simulink model "MPC2018a"  (R2019b)
settings: Solver=FixedStepAuto  StartTime=0.0  StopTime=80  FixedStep=0.05  RelTol=1e-3
InitFcn:
  | startPose=[0,0,48]
StopFcn:
  | load('NewBaiYunPathDown6_13.mat')
  | n=1;
  | x0=0;
  | y0=0;
  | lng0 = BaiYunEmpty(2,1);
  | lat0 = BaiYunEmpty(1,1);
  | x1=[];
  | y1=[];
  | head=[];
  | nn = length(BaiYunEmpty(1,:));
  | while (n<nn)
  | lng2 = BaiYunEmpty(2,n);
  | lat2 = BaiYunEmpty(1,n);
  | head2 = BaiYunEmpty(3,n);
  | temp_x=(lng2-lng0)*111700*cos(lat2/180*pi);
  | temp_y=(lat2-lat0)*111700;
  | x1(n) = x0 + temp_x;
  | y1(n) = y0 + temp_y;
  | head(n)=head2;
  | n = n+1;
  | end
  | figure(1);
  | plot(x1,y1,'+r',out.v2(:,1),out.v2(:,2),'+k',out.v3(:,1),out.v3(:,2),'+b');
libraries: simulink x21, simulink_extras x4, drivingvehiclecontroller x2, vehdynlibsteering x2, autolibshared x2
(part 1 of 2)
settings Model: NumberOfSteps=10  SnapshotBufferSize=100  Creator=hurui  LastModifiedBy=HL
settings SolverCC: AlgebraicLoopSolver=LineSearch
settings DataIOCC: SaveFormat=StructureWithTime
settings OptimizationCC: BlockReduction=off  UseDivisionForNetSlopeComputation=on  BufferReuse=off
settings DebuggingCC: AlgebraicLoopMsg=none  UnconnectedInputMsg=none  UnconnectedOutputMsg=none  UnconnectedLineMsg=none  UnderSpecifiedDimensionMsg=warning
settings SFSimCC: SimParseCustomCode=off

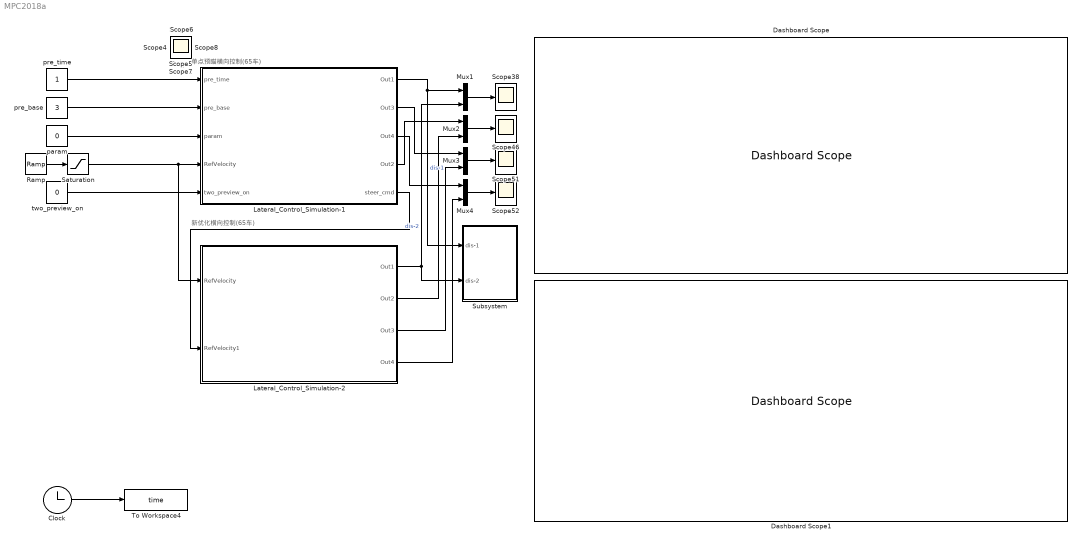
== system MPC2018a ==
  note: 单点预瞄横向控制(65车)
  note: 新优化横向控制(65车)
  Clock : Clock
  Dashboard Scope : DashboardScope
  Dashboard Scope1 : DashboardScope
  Lateral_Control_Simulation-1 : Subsystem
  Lateral_Control_Simulation-2 : Subsystem
  Mux{1..4} (4 alike) : Mux  Inputs=2
  Ramp : simulink/Sources/Ramp  slope=1  start=0  InitialOutput=0
  Saturation : Saturate  UpperLimit=15  LowerLimit=0
  Scope{,1..8,38,46,51..52} (13 alike) : Scope
  Subsystem : Subsystem
  To Workspace4 : ToWorkspace  VariableName=time  SampleTime=-1
      settings: Save2DSignal=2-D array (concatenate along first dimension)
  param : Constant  Value=0  OutDataTypeStr=single
  pre_base : Constant  Value=3  OutDataTypeStr=single
  pre_time : Constant  OutDataTypeStr=single
  two_preview_on : Constant  Value=0  OutDataTypeStr=single
  wires:
  Lateral_Control_Simulation-1/1(Out1) -> Subsystem/1(dis-1), Mux1/1  "dis-1"
  Lateral_Control_Simulation-2/1(Out1) -> Mux1/2, Subsystem/2(dis-2)  "dis-2"
  Mux1/1 -> Scope38/1
  Lateral_Control_Simulation-1/4(Out2) -> Mux2/1
  Lateral_Control_Simulation-2/2(Out2) -> Mux2/2
  Mux2/1 -> Scope46/1
  pre_time/1 -> Lateral_Control_Simulation-1/1(pre_time)
  pre_base/1 -> Lateral_Control_Simulation-1/2(pre_base)
  param/1 -> Lateral_Control_Simulation-1/3(param)
  Saturation/1 -> Lateral_Control_Simulation-1/4(RefVelocity), Lateral_Control_Simulation-2/1(RefVelocity)
  two_preview_on/1 -> Lateral_Control_Simulation-1/5(two_preview_on)
  Clock/1 -> To Workspace4/1
  Ramp/1 -> Saturation/1
  Lateral_Control_Simulation-1/2(Out3) -> Mux3/1
  Lateral_Control_Simulation-2/3(Out3) -> Mux3/2
  Lateral_Control_Simulation-1/3(Out4) -> Mux4/1
  Lateral_Control_Simulation-2/4(Out4) -> Mux4/2
  Mux3/1 -> Scope51/1
  Mux4/1 -> Scope52/1
  Lateral_Control_Simulation-1/5(steer_cmd) -> Lateral_Control_Simulation-2/2(RefVelocity1)

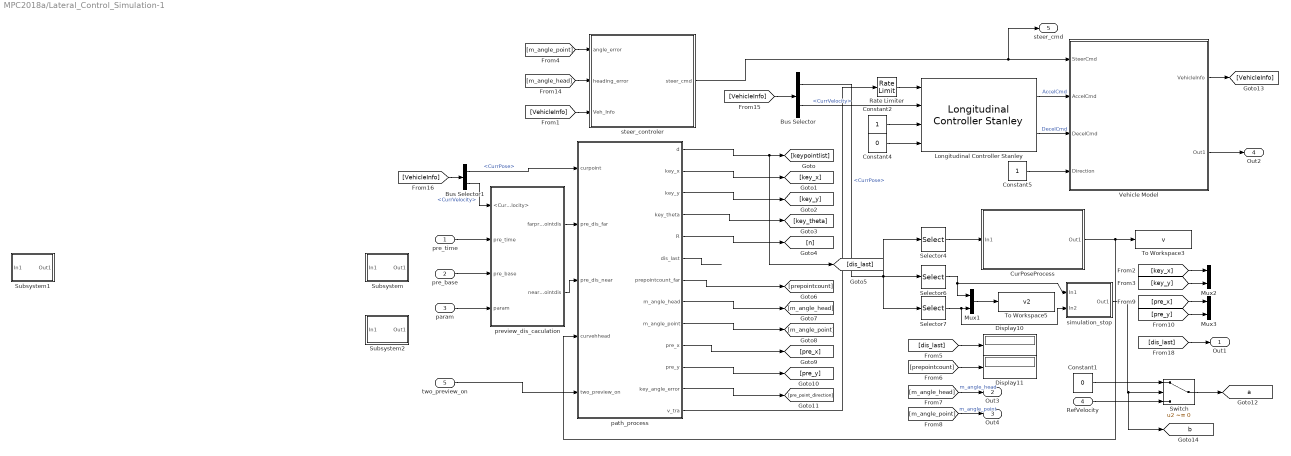
== system MPC2018a/Lateral_Control_Simulation-1 ==
  pre_time : Inport
  pre_base : Inport  Port=2
  param : Inport  Port=3
  RefVelocity : Inport  Port=4
  two_preview_on : Inport  Port=5
  Bus Selector : BusSelector  OutputSignals=CurrPose,CurrVelocity
  Bus Selector1 : BusSelector  OutputSignals=CurrPose,CurrVelocity
  Constant1 : Constant  Value=0
  Constant2 : Constant
  Constant4 : Constant  Value=0
  Constant5 : Constant
  CurPoseProcess : Subsystem
  Display10 : Display
  Display11 : Display
  Longitudinal Controller Stanley : drivingvehiclecontroller/Longitudinal Controller Stanley  Kp=2.5  Ki=1  SampleTime=0.05  MaxAcceleration=3  MaxDeceleration=25
      settings: SourceProductBaseCode=DR
  Mux1 : Mux  Inputs=2
  Mux2 : Mux  Inputs=2
  Mux3 : Mux  Inputs=2
  Rate Limiter : RateLimiter  SampleTimeMode=inherited
  Selector4 : Selector  InputPortWidth=3  IndexOptions=Index vector (dialog)  Indices=[3]  OutputSizes=1
  Selector6 : Selector  InputPortWidth=3  IndexOptions=Index vector (dialog)  Indices=[1]  OutputSizes=1
  Selector7 : Selector  InputPortWidth=3  IndexOptions=Index vector (dialog)  Indices=[2]  OutputSizes=1
  Subsystem : Subsystem
  Subsystem1 : Subsystem
  Subsystem2 : Subsystem
  Switch : Switch  Criteria=u2 ~= 0
  To Workspace3 : ToWorkspace  VariableName=v  SampleTime=-1
      settings: Save2DSignal=2-D array (concatenate along first dimension)
  To Workspace5 : ToWorkspace  VariableName=v2  SampleTime=-1
      settings: Save2DSignal=2-D array (concatenate along first dimension)
  Vehicle Model : Subsystem
  path_process : MATLAB Function  TreatAsAtomicUnit=on  VariantControl=(default)
  preview_dis_caculation : Subsystem
  simulation_stop : Subsystem
  steer_controler : Subsystem
  Out1 : Outport
  Out3 : Outport  Port=2
  Out4 : Outport  Port=3
  Out2 : Outport  Port=4
  steer_cmd : Outport  Port=5
  tag scope: a=global, b=global
  wires:
  pre_time/1 -> preview_dis_caculation/2(pre_time)
  pre_base/1 -> preview_dis_caculation/3(pre_base)
  param/1 -> preview_dis_caculation/4(param)
  [dis_last] -> Out1/1
  path_process/8(m_angle_head) -> [m_angle_head]
  Bus Selector/1 -> Selector4/1, Selector7/1, Selector6/1  "<CurrPose>"
  [VehicleInfo] -> Bus Selector1/1
  Mux1/1 -> To Workspace5/1
  Constant2/1 -> Longitudinal Controller Stanley/3
  path_process/6(dis_last) -> ?
  preview_dis_caculation/1(farprepointdis) -> path_process/2(pre_dis_far)
  Longitudinal Controller Stanley/2 -> Vehicle Model/3(DecelCmd)  "DecelCmd"
  Bus Selector/2 -> Longitudinal Controller Stanley/2  "<CurrVelocity>"
  path_process/4(key_theta) -> [key_theta]
  [VehicleInfo] -> steer_controler/3(Veh_Info)
  Bus Selector1/1 -> path_process/1(curpoint)  "<CurrPose>"
  Selector6/1 -> Mux1/1, simulation_stop/1(In1)
  Constant4/1 -> Longitudinal Controller Stanley/4
  Constant5/1 -> Vehicle Model/4(Direction)
  preview_dis_caculation/2(nearprepointdis) -> path_process/3(pre_dis_near)
  [m_angle_head] -> Out3/1  "m_angle_head"
  path_process/7(prepointcount_far) -> [prepointcount]
  Selector7/1 -> simulation_stop/2(In2), Mux1/2
  path_process/12(key_angle_error) -> [pre_point_direction]
  path_process/10(pre_x) -> [pre_x]
  path_process/2(key_x) -> [key_x]
  [pre_y] -> Mux3/2
  steer_controler/1(steer_cmd) -> steer_cmd/1, Vehicle Model/1(SteerCmd)
  [key_x] -> Mux2/1
  Longitudinal Controller Stanley/1 -> Vehicle Model/2(AccelCmd)  "AccelCmd"
  path_process/3(key_y) -> [key_y]
  Bus Selector1/2 -> preview_dis_caculation/1(<CurrVelocity>)  "<CurrVelocity>"
  path_process/9(m_angle_point) -> [m_angle_point]
  [VehicleInfo] -> Bus Selector/1
  [pre_x] -> Mux3/1
  [key_y] -> Mux2/2
  [m_angle_head] -> steer_controler/2(heading_error)
  [dis_last] -> Display10/1
  [m_angle_point] -> Out4/1  "m_angle_point"
  [m_angle_point] -> steer_controler/1(angle_error)
  path_process/11(pre_y) -> [pre_y]
  [prepointcount] -> Display11/1
  path_process/5(R) -> [n]
  Vehicle Model/1(VehicleInfo) -> [VehicleInfo]
  RefVelocity/1 -> Switch/3
  Selector4/1 -> CurPoseProcess/1(In1)
  CurPoseProcess/1(Out1) -> path_process/4(curvehhead), To Workspace3/1
  two_preview_on/1 -> path_process/5(two_preview_on)
  Vehicle Model/2(Out1) -> Out2/1
  simulation_stop/1(Out1) -> [b], Switch/2
  Constant1/1 -> Switch/1
  Switch/1 -> [a]
  Rate Limiter/1 -> Longitudinal Controller Stanley/1
  path_process/13(v_tra) -> Rate Limiter/1
  path_process/1(d) -> [dis_last], [keypointlist]

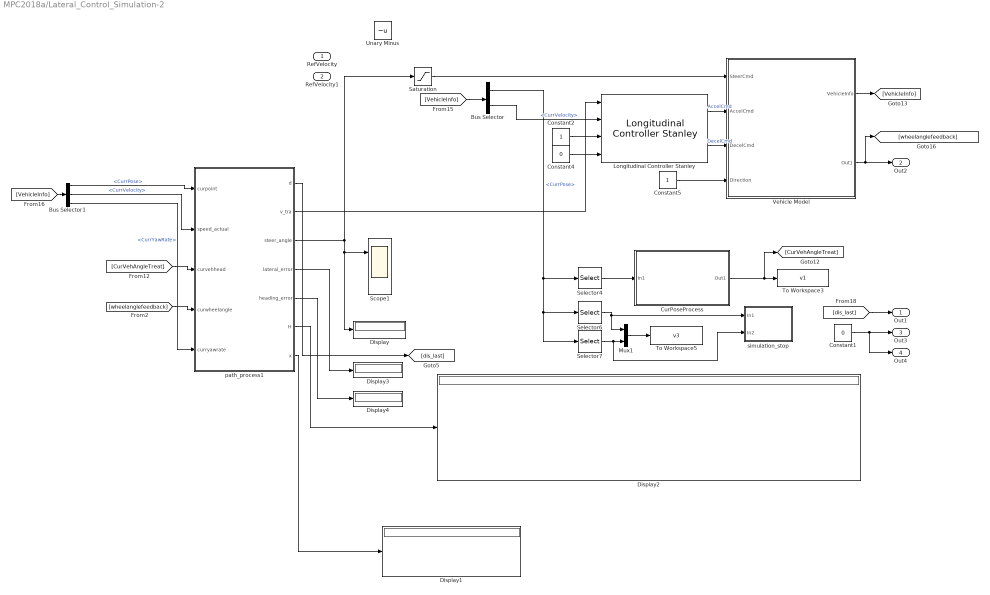
== system MPC2018a/Lateral_Control_Simulation-2 ==
  RefVelocity : Inport
  RefVelocity1 : Inport  Port=2
  Bus Selector : BusSelector  OutputSignals=CurrPose,CurrVelocity
  Bus Selector1 : BusSelector  OutputSignals=CurrPose,CurrVelocity,CurrYawRate
  Constant1 : Constant  Value=0
  Constant2 : Constant
  Constant4 : Constant  Value=0
  Constant5 : Constant  SampleTime=-1
  CurPoseProcess : Subsystem
  Display{,1..4} (5 alike) : Display
  Longitudinal Controller Stanley : drivingvehiclecontroller/Longitudinal Controller Stanley  Kp=2.5  Ki=1  SampleTime=0.05  MaxAcceleration=3  MaxDeceleration=5
      settings: SourceProductBaseCode=DR
  Mux1 : Mux  Inputs=2
  Saturation : Saturate  UpperLimit=30  LowerLimit=-30
  Scope1 : Scope  NumInputPorts=2
  Selector4 : Selector  InputPortWidth=3  IndexOptions=Index vector (dialog)  Indices=[3]  OutputSizes=1
  Selector6 : Selector  InputPortWidth=3  IndexOptions=Index vector (dialog)  Indices=[1]  OutputSizes=1
  Selector7 : Selector  InputPortWidth=3  IndexOptions=Index vector (dialog)  Indices=[2]  OutputSizes=1
  To Workspace3 : ToWorkspace  VariableName=v1  SampleTime=-1
      settings: Save2DSignal=2-D array (concatenate along first dimension)
  To Workspace5 : ToWorkspace  VariableName=v3  SampleTime=-1
      settings: Save2DSignal=2-D array (concatenate along first dimension)
  Unary Minus : UnaryMinus
  Vehicle Model : Subsystem
  path_process1 : MATLAB Function  Priority=1  TreatAsAtomicUnit=on  VariantControl=(default)
  simulation_stop : Subsystem
  Out1 : Outport
  Out2 : Outport  Port=2
  Out3 : Outport  Port=3
  Out4 : Outport  Port=4
  wires:
  CurPoseProcess/1(Out1) -> [CurVehAngleTreat], To Workspace3/1
  Selector4/1 -> CurPoseProcess/1(In1)
  Vehicle Model/1(VehicleInfo) -> [VehicleInfo]
  Constant1/1 -> Out4/1, Out3/1
  [VehicleInfo] -> Bus Selector/1
  Longitudinal Controller Stanley/1 -> Vehicle Model/2(AccelCmd)  "AccelCmd"
  Selector7/1 -> simulation_stop/2(In2), Mux1/2
  Constant5/1 -> Vehicle Model/4(Direction)
  Constant4/1 -> Longitudinal Controller Stanley/4
  Selector6/1 -> Mux1/1, simulation_stop/1(In1)
  Bus Selector/2 -> Longitudinal Controller Stanley/2  "<CurrVelocity>"
  Longitudinal Controller Stanley/2 -> Vehicle Model/3(DecelCmd)  "DecelCmd"
  Constant2/1 -> Longitudinal Controller Stanley/3
  Mux1/1 -> To Workspace5/1
  [VehicleInfo] -> Bus Selector1/1
  Bus Selector/1 -> Selector6/1, Selector7/1, Selector4/1  "<CurrPose>"
  [dis_last] -> Out1/1
  Vehicle Model/2(Out1) -> [wheelanglefeedback], Out2/1
  path_process1/1(d) -> [dis_last]
  [CurVehAngleTreat] -> path_process1/3(curvehhead)
  [wheelanglefeedback] -> path_process1/4(curwheelangle)
  Bus Selector1/1 -> path_process1/1(curpoint)  "<CurrPose>"
  Bus Selector1/2 -> path_process1/2(speed_actual)  "<CurrVelocity>"
  Bus Selector1/3 -> path_process1/5(curryawrate)  "<CurrYawRate>"
  path_process1/2(v_tra) -> Longitudinal Controller Stanley/1
  Saturation/1 -> Vehicle Model/1(SteerCmd)
  path_process1/4(lateral_error) -> Display3/1
  path_process1/3(steer_angle) -> Display/1, Scope1/1, Saturation/1
  path_process1/5(heading_error) -> Display4/1
  path_process1/6(H) -> Display2/1
  path_process1/7(x) -> Display1/1

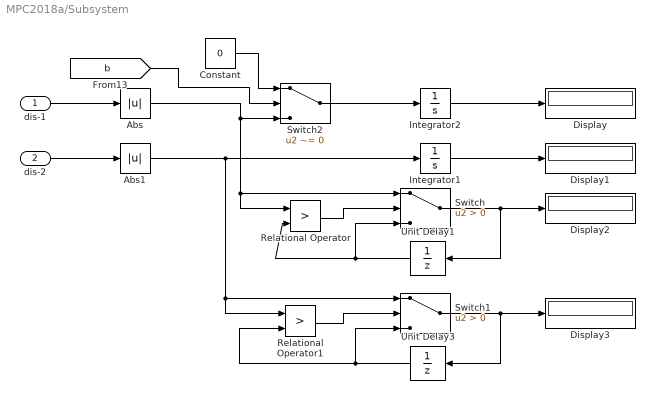
== system MPC2018a/Subsystem ==
  dis-1 : Inport
  dis-2 : Inport  Port=2
  Abs : Abs
  Abs1 : Abs
  Constant : Constant  Value=0
  Display{,1..3} (4 alike) : Display
  Integrator1 : Integrator
  Integrator2 : Integrator
  Relational Operator : RelationalOperator  Operator=>  OutDataTypeStr=boolean  RndMeth=Simplest
  Relational Operator1 : RelationalOperator  Operator=>  OutDataTypeStr=boolean  RndMeth=Simplest
  Switch : Switch  Criteria=u2 > Threshold
  Switch1 : Switch  Criteria=u2 > Threshold
  Switch2 : Switch  Criteria=u2 ~= 0
  Unit Delay1 : UnitDelay  SampleTime=-1  HasFrameUpgradeWarning=on
  Unit Delay3 : UnitDelay  SampleTime=-1  HasFrameUpgradeWarning=on
  wires:
  Integrator1/1 -> Display1/1
  Switch1/1 -> Unit Delay3/1, Display3/1
  Unit Delay3/1 -> Relational Operator1/2, Switch1/3
  Abs/1 -> Switch2/3, Switch/1, Relational Operator/1
  Abs1/1 -> Relational Operator1/1, Switch1/1, Integrator1/1
  Unit Delay1/1 -> Switch/3, Relational Operator/2
  Relational Operator1/1 -> Switch1/2
  Relational Operator/1 -> Switch/2
  Switch/1 -> Unit Delay1/1, Display2/1
  dis-1/1 -> Abs/1
  dis-2/1 -> Abs1/1
  [b] -> Switch2/2
  Constant/1 -> Switch2/1
  Switch2/1 -> Integrator2/1
  Integrator2/1 -> Display/1

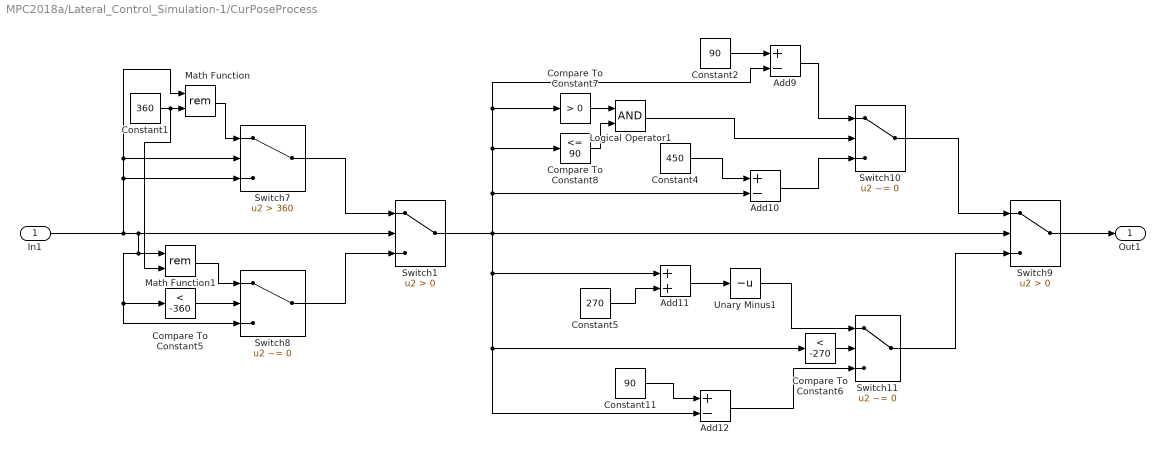
== system MPC2018a/Lateral_Control_Simulation-1/CurPoseProcess ==
  In1 : Inport
  Add10 : Sum  Inputs=+-
  Add11 : Sum
  Add12 : Sum  Inputs=+-
  Add9 : Sum  Inputs=+-
  Compare To Constant5 : simulink/Logic and Bit Operations/Compare To Constant  relop=<  const=-360  OutDataTypeStr=boolean
  Compare To Constant6 : simulink/Logic and Bit Operations/Compare To Constant  relop=<  const=-270  OutDataTypeStr=boolean
  Compare To Constant7 : simulink/Logic and Bit Operations/Compare To Constant  relop=>  const=0  OutDataTypeStr=boolean
  Compare To Constant8 : simulink/Logic and Bit Operations/Compare To Constant  relop=<=  const=90  OutDataTypeStr=boolean
  Constant1 : Constant  Value=360
  Constant11 : Constant  Value=90
  Constant2 : Constant  Value=90
  Constant4 : Constant  Value=450
  Constant5 : Constant  Value=270
  Logical Operator1 : Logic  AllPortsSameDT=off  OutDataTypeStr=boolean
  Math Function : Math  Operator=rem  SignedPower=off  SaturateOnIntegerOverflow=on
  Math Function1 : Math  Operator=rem  SignedPower=off  SaturateOnIntegerOverflow=on
  Switch1 : Switch  Criteria=u2 > Threshold
  Switch10 : Switch  Criteria=u2 ~= 0  Threshold=360
  Switch11 : Switch  Criteria=u2 ~= 0  Threshold=360
  Switch7 : Switch  Criteria=u2 > Threshold  Threshold=360
  Switch8 : Switch  Criteria=u2 ~= 0  Threshold=360
  Switch9 : Switch  Criteria=u2 > Threshold
  Unary Minus1 : UnaryMinus
  Out1 : Outport
  wires:
  In1/1 -> Switch1/2, Switch8/3, Compare To Constant5/1, Math Function1/1, Math Function/1, Switch7/2, Switch7/3
  Switch7/1 -> Switch1/1
  Math Function/1 -> Switch7/1
  Constant1/1 -> Math Function1/2, Math Function/2
  Switch8/1 -> Switch1/3
  Compare To Constant5/1 -> Switch8/2
  Math Function1/1 -> Switch8/1
  Switch1/1 -> Add11/1, Add12/2, Compare To Constant6/1, Add9/2, Compare To Constant7/1, Compare To Constant8/1, Add10/2, Switch9/2
  Switch10/1 -> Switch9/1
  Add9/1 -> Switch10/1
  Constant2/1 -> Add9/1
  Add10/1 -> Switch10/3
  Constant4/1 -> Add10/1
  Compare To Constant6/1 -> Switch11/2
  Add11/1 -> Unary Minus1/1
  Constant5/1 -> Add11/2
  Unary Minus1/1 -> Switch11/1
  Add12/1 -> Switch11/3
  Constant11/1 -> Add12/1
  Switch11/1 -> Switch9/3
  Switch9/1 -> Out1/1
  Compare To Constant7/1 -> Logical Operator1/1
  Compare To Constant8/1 -> Logical Operator1/2
  Logical Operator1/1 -> Switch10/2

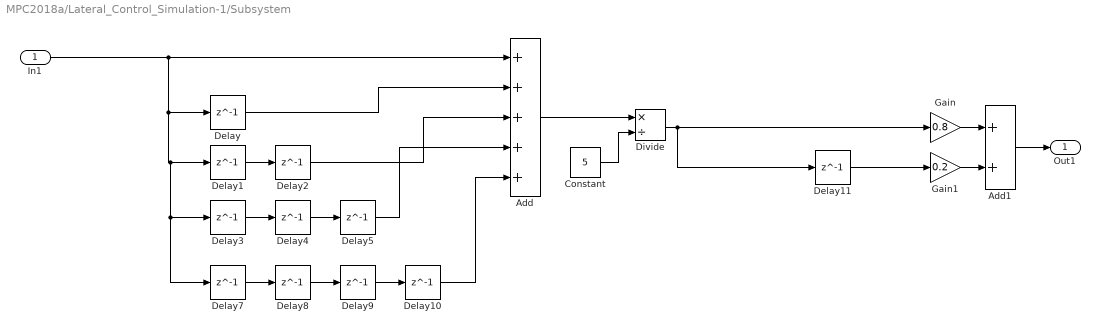
== system MPC2018a/Lateral_Control_Simulation-1/Subsystem ==
  In1 : Inport
  Add : Sum  Inputs=+++++
  Add1 : Sum
  Constant : Constant  Value=5
  Delay{,1..5,7..11} (11 alike) : Delay  DelayLength=1  InitialCondition=0
  Divide : Product  Inputs=*/
  Gain : Gain  Gain=0.8
  Gain1 : Gain  Gain=0.2
  Out1 : Outport
  wires:
  Delay10/1 -> Add/5
  Delay5/1 -> Add/4
  In1/1 -> Add/1, Delay3/1, Delay7/1, Delay1/1, Delay/1
  Delay1/1 -> Delay2/1
  Delay3/1 -> Delay4/1
  Delay4/1 -> Delay5/1
  Delay/1 -> Add/2
  Delay2/1 -> Add/3
  Add/1 -> Divide/1
  Constant/1 -> Divide/2
  Gain/1 -> Add1/1
  Gain1/1 -> Add1/2
  Add1/1 -> Out1/1
  Divide/1 -> Gain/1, Delay11/1
  Delay8/1 -> Delay9/1
  Delay7/1 -> Delay8/1
  Delay9/1 -> Delay10/1
  Delay11/1 -> Gain1/1

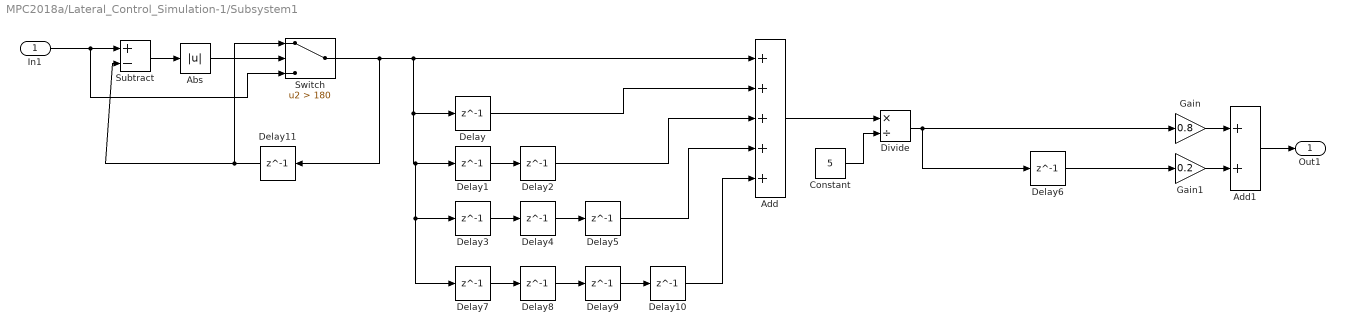
== system MPC2018a/Lateral_Control_Simulation-1/Subsystem1 ==
  In1 : Inport
  Abs : Abs
  Add : Sum  Inputs=+++++
  Add1 : Sum
  Constant : Constant  Value=5
  Delay{,1..11} (12 alike) : Delay  DelayLength=1  InitialCondition=0
  Divide : Product  Inputs=*/
  Gain : Gain  Gain=0.8
  Gain1 : Gain  Gain=0.2
  Subtract : Sum  Inputs=+-
  Switch : Switch  Criteria=u2 > Threshold  Threshold=180
  Out1 : Outport
  wires:
  Delay6/1 -> Gain1/1
  Delay10/1 -> Add/5
  Delay9/1 -> Delay10/1
  Delay7/1 -> Delay8/1
  Delay8/1 -> Delay9/1
  Add1/1 -> Out1/1
  Gain1/1 -> Add1/2
  Gain/1 -> Add1/1
  Divide/1 -> Delay6/1, Gain/1
  Constant/1 -> Divide/2
  Add/1 -> Divide/1
  Delay5/1 -> Add/4
  Delay2/1 -> Add/3
  Delay/1 -> Add/2
  Delay4/1 -> Delay5/1
  Delay3/1 -> Delay4/1
  Delay1/1 -> Delay2/1
  Switch/1 -> Delay11/1, Delay/1, Delay1/1, Delay7/1, Delay3/1, Add/1
  Delay11/1 -> Switch/1, Subtract/2
  In1/1 -> Switch/3, Subtract/1
  Subtract/1 -> Abs/1
  Abs/1 -> Switch/2

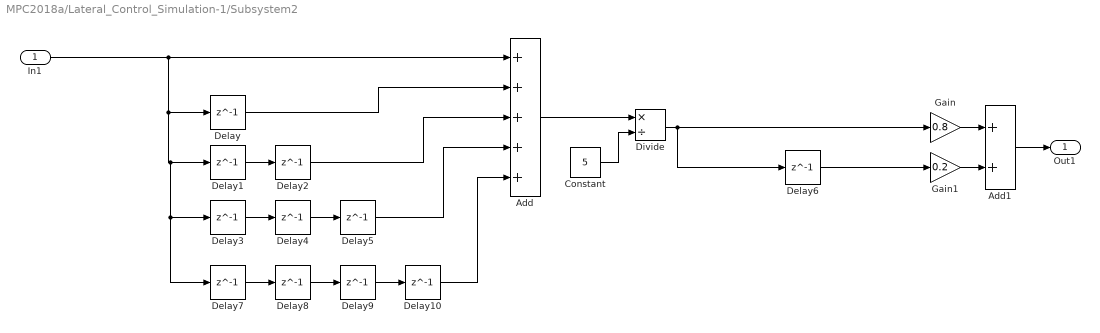
== system MPC2018a/Lateral_Control_Simulation-1/Subsystem2 ==
  In1 : Inport
  Add : Sum  Inputs=+++++
  Add1 : Sum
  Constant : Constant  Value=5
  Delay{,1..10} (11 alike) : Delay  DelayLength=1  InitialCondition=0
  Divide : Product  Inputs=*/
  Gain : Gain  Gain=0.8
  Gain1 : Gain  Gain=0.2
  Out1 : Outport
  wires:
  In1/1 -> Add/1, Delay3/1, Delay7/1, Delay1/1, Delay/1
  Delay1/1 -> Delay2/1
  Delay3/1 -> Delay4/1
  Delay4/1 -> Delay5/1
  Delay/1 -> Add/2
  Delay2/1 -> Add/3
  Delay5/1 -> Add/4
  Add/1 -> Divide/1
  Constant/1 -> Divide/2
  Divide/1 -> Gain/1, Delay6/1
  Gain/1 -> Add1/1
  Gain1/1 -> Add1/2
  Add1/1 -> Out1/1
  Delay8/1 -> Delay9/1
  Delay7/1 -> Delay8/1
  Delay9/1 -> Delay10/1
  Delay10/1 -> Add/5
  Delay6/1 -> Gain1/1

== system MPC2018a/Lateral_Control_Simulation-1/Vehicle Model ==
  SteerCmd : Inport
  AccelCmd : Inport  Port=2
  DecelCmd : Inport  Port=3
  Direction : Inport  Port=4
  Acceleration to Velocity : Subsystem  TreatAsAtomicUnit=on
  Constant5 : Constant  Value=4  SampleTime=-1
  Degrees to Radians : simulink_extras/Transformations/Degrees to Radians
  Delayed Steering System : Subsystem
  Kinematic Steering : vehdynlibsteering/Kinematic Steering  StrgType=Ackerman  StrgRatioType=Constant  Loc=Front  NrmlFctr=1  TrckWdth=2.35  WhlBase=5.275  Db=0  StrgRng=1.25*pi  StrgAngBpts="[-6.2832   -5.0265   -3.7699   -2.5133   -1.2566         0    1.2566    2.5133    3.7699    5.0265    6.2832]"  StrgRatioTbl=|  StrgRatio=1  StrgArmLngth=0.1  RckCsLngth=0.5  TieRodLngth=0.248  D=0.2  PnnRadius=0.0057  PnnRadiusTbl="[0.0055    0.0055    0.0056    0.0057    0.0058    0.0057    0.0057    0.0057    0.0056    0.0055    0.0055]"  RodLngth=0.1  ParaArmLngth=0.9  aMode=2
      | [13.5000   13.3750   13.2500   13.1250   13.0000   13.0000   13.0000   13.1250   13.2500   13.3750   13.5000
      | ]
  Mux : Mux  Inputs=2
  Subsystem : Subsystem
  Terminator : Terminator
  Terminator1 : Terminator
  Terminator2 : Terminator
  Vehicle Body 3DOF Dual Track : autolibshared/Vehicle Body 3DOF Single Track  trackMode=Dual  inputMode=External longitudinal velocity  frontSteerMode=on  rearSteerMode=off  windMode=off  muMode=off  extFMode=off  extMMode=off  extXo=off  extpsio=off  extxdoto=off  extro=off  extYo=off  extTamb=off  extydoto=off  aMode=2  NF=2  NR=4  m=25000  a=2.55  b=2.675  h=0.8  X_o=startPose(1)+cosd(startPose(3))*1.6  xdot_o=0  CalphaMode=off  sigmaMode=off  d=0  w=[2.35,2.6]  Cy_f=4e4  Cy_r=6e4  sigma_f=.1  sigma_r=.1  alpha_f_brk=[-.1 .1]  Cy_f_data=[-9e3 9e3]  alpha_r_brk=[-.1 .1]  Cy_r_data=[-9e3 9e3]  Y_o=startPose(2) +sind(startPose(3))*1.6  ydot_o=0  Izz=60000  psi_o=deg2rad(startPose(3))  r_o=0  Af=6  Cd=.3  Cl=0  Cpm=.1  beta_w=[0:0.01:0.3]  Cs=[0:0.03:0.9]  Cym=[0:0.01:0.3]  Pabs=101325  Tair=273  g=9.81  mu=1  xdot_tol=.01  Fznom=5000  Fxtire_sat=7e4  Fytire_sat=7e4  longOff=0  latOff=0  vertOff=0  wrapAng=off
      settings: SourceProductBaseCode=PW,MT,VE,VP
  VehicleInfo : Outport  VectorParamsAs1DForOutWhenUnconnected=off
  Out1 : Outport  Port=2
  wires:
  Direction/1 -> Acceleration to Velocity/3(Direction), Subsystem/7(<Direction>)
  SteerCmd/1 -> Delayed Steering System/1(SteerCmd)  "CurrSteer"
  DecelCmd/1 -> Acceleration to Velocity/2(DecelCmd)
  AccelCmd/1 -> Acceleration to Velocity/1(AccelCmd)
  Subsystem/1(VehicleInfo) -> VehicleInfo/1
  Vehicle Body 3DOF Dual Track/1 -> Subsystem/2(Info)
  Vehicle Body 3DOF Dual Track/2 -> Subsystem/3(In3)
  Vehicle Body 3DOF Dual Track/3 -> Subsystem/4(In4)
  Vehicle Body 3DOF Dual Track/4 -> Subsystem/5(In5)
  Vehicle Body 3DOF Dual Track/5 -> Subsystem/6(In6)
  Vehicle Body 3DOF Dual Track/6 -> Terminator/1
  Vehicle Body 3DOF Dual Track/7 -> Terminator1/1
  Kinematic Steering/1 -> Terminator2/1
  Kinematic Steering/2 -> Mux/1
  Kinematic Steering/3 -> Mux/2
  Degrees to Radians/1 -> Kinematic Steering/1
  Delayed Steering System/1(CurrSteer) -> Out1/1, Subsystem/1(CurrSteer), Degrees to Radians/1  "CurrSteer"
  Mux/1 -> Vehicle Body 3DOF Dual Track/1
  Constant5/1 -> Vehicle Body 3DOF Dual Track/2

== system MPC2018a/Lateral_Control_Simulation-1/preview_dis_caculation ==
  <CurrVelocity> : Inport
  pre_time : Inport  Port=2
  pre_base : Inport  Port=3
  param : Inport  Port=4
  far_pre_dis caculaiton : Subsystem
  near_pre_dis caculaiton : Subsystem
  farprepointdis : Outport
  nearprepointdis : Outport  Port=2
  wires:
  param/1 -> far_pre_dis caculaiton/4(param)
  pre_base/1 -> far_pre_dis caculaiton/3(pre_base)
  pre_time/1 -> far_pre_dis caculaiton/2(pre_time)
  <CurrVelocity>/1 -> near_pre_dis caculaiton/1(vehiclespeed), far_pre_dis caculaiton/1(vehiclespeed)
  near_pre_dis caculaiton/1(nearprepointdis) -> nearprepointdis/1
  far_pre_dis caculaiton/1(farprepointdis) -> farprepointdis/1

== system MPC2018a/Lateral_Control_Simulation-1/simulation_stop ==
  In1 : Inport
  In2 : Inport  Port=2
  Compare To Constant : simulink/Logic and Bit Operations/Compare To Constant  relop=<=  const=-320  OutDataTypeStr=boolean
  Compare To Constant1 : simulink/Logic and Bit Operations/Compare To Constant  relop=>=  const=-340  OutDataTypeStr=boolean
  Compare To Constant2 : simulink/Logic and Bit Operations/Compare To Constant  relop=<=  const=240  OutDataTypeStr=boolean
  Compare To Constant3 : simulink/Logic and Bit Operations/Compare To Constant  relop=>=  const=220  OutDataTypeStr=boolean
  Logical Operator : Logic  AllPortsSameDT=off  OutDataTypeStr=boolean
  Logical Operator1 : Logic  AllPortsSameDT=off  OutDataTypeStr=boolean
  Logical Operator2 : Logic  AllPortsSameDT=off  OutDataTypeStr=boolean
  Stop Simulation : Stop
  Out1 : Outport
  wires:
  Compare To Constant/1 -> Logical Operator/1
  In1/1 -> Compare To Constant/1, Compare To Constant1/1
  Compare To Constant1/1 -> Logical Operator/2
  Logical Operator/1 -> Logical Operator1/1
  Logical Operator2/1 -> Logical Operator1/2
  Compare To Constant2/1 -> Logical Operator2/1
  Compare To Constant3/1 -> Logical Operator2/2
  In2/1 -> Compare To Constant3/1, Compare To Constant2/1
  Logical Operator1/1 -> Stop Simulation/1, Out1/1

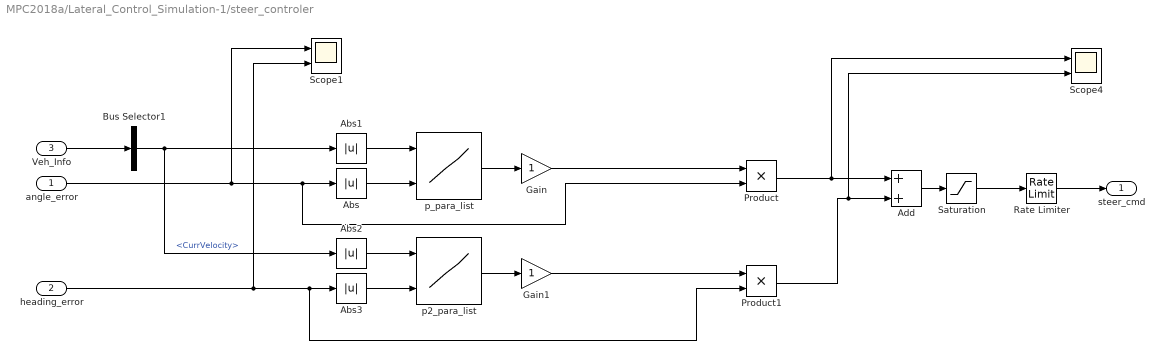
== system MPC2018a/Lateral_Control_Simulation-1/steer_controler ==
  angle_error : Inport
  heading_error : Inport  Port=2
  Veh_Info : Inport  Port=3
  Abs{,1..3} (4 alike) : Abs
  Add : Sum
  Bus Selector1 : BusSelector  OutputSignals=CurrVelocity
  Gain : Gain
  Gain1 : Gain
  Product : Product
  Product1 : Product
  Rate Limiter : RateLimiter  RisingSlewLimit=28  FallingSlewLimit=-28  SampleTimeMode=inherited
  Saturation : Saturate  UpperLimit=35  LowerLimit=-35
  Scope1 : Scope  NumInputPorts=2
  Scope4 : Scope  NumInputPorts=2
  p2_para_list : Lookup_n-D  BreakpointsForDimension1=[0,7,15,22,30]  BreakpointsForDimension2=[0,5,12,20,30]  Table=reshape([0.2,0.2,0.2,0.2,0.2,0.3,0.3,0.2,0.2,0.2,0.3,0.3,0.2,0.2,0.2,0.3,0.3,0.3,0.2,0.2,0.4,0.3,0.3,0.2,0.2],5,5)  ExtrapMethod=Clip  InternalRulePriority=Speed  RndMeth=Simplest  InputSameDT=on
  p_para_list : Lookup_n-D  BreakpointsForDimension1=[0,7,15,22,30]  BreakpointsForDimension2=[0,5,12,20,30]  Table=reshape([0.4,0.4,0.4,0.4,0.3,0.4,0.4,0.4,0.4,0.3,0.5,0.5,0.4,0.4,0.3,0.5,0.5,0.4,0.4,0.3,0.5,0.5,0.4,0.4,0.3],5,5)  ExtrapMethod=Clip  InternalRulePriority=Speed  RndMeth=Simplest  InputSameDT=on
  steer_cmd : Outport
  wires:
  p_para_list/1 -> Gain/1
  p2_para_list/1 -> Gain1/1
  Product/1 -> Scope4/1, Add/1
  Product1/1 -> Scope4/2, Add/2
  Gain/1 -> Product/1
  Gain1/1 -> Product1/1
  Veh_Info/1 -> Bus Selector1/1
  Abs1/1 -> p_para_list/1
  Abs/1 -> p_para_list/2
  Bus Selector1/1 -> Abs2/1, Abs1/1  "<CurrVelocity>"
  angle_error/1 -> Scope1/1, Product/2, Abs/1
  heading_error/1 -> Scope1/2, Abs3/1, Product1/2
  Abs2/1 -> p2_para_list/1
  Abs3/1 -> p2_para_list/2
  Add/1 -> Saturation/1
  Saturation/1 -> Rate Limiter/1
  Rate Limiter/1 -> steer_cmd/1

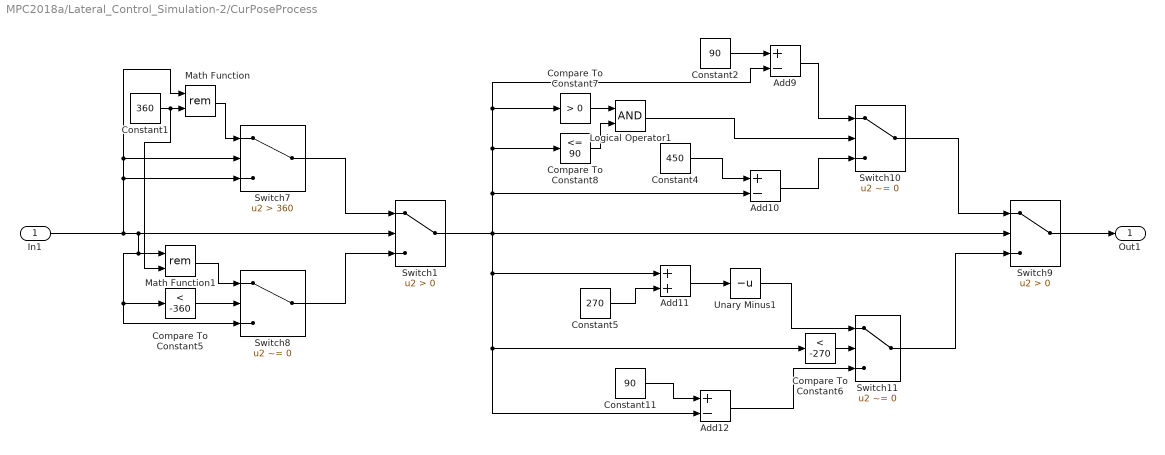
== system MPC2018a/Lateral_Control_Simulation-2/CurPoseProcess ==
  In1 : Inport
  Add10 : Sum  Inputs=+-
  Add11 : Sum
  Add12 : Sum  Inputs=+-
  Add9 : Sum  Inputs=+-
  Compare To Constant5 : simulink/Logic and Bit Operations/Compare To Constant  relop=<  const=-360  OutDataTypeStr=boolean
  Compare To Constant6 : simulink/Logic and Bit Operations/Compare To Constant  relop=<  const=-270  OutDataTypeStr=boolean
  Compare To Constant7 : simulink/Logic and Bit Operations/Compare To Constant  relop=>  const=0  OutDataTypeStr=boolean
  Compare To Constant8 : simulink/Logic and Bit Operations/Compare To Constant  relop=<=  const=90  OutDataTypeStr=boolean
  Constant1 : Constant  Value=360
  Constant11 : Constant  Value=90
  Constant2 : Constant  Value=90
  Constant4 : Constant  Value=450
  Constant5 : Constant  Value=270
  Logical Operator1 : Logic  AllPortsSameDT=off  OutDataTypeStr=boolean
  Math Function : Math  Operator=rem  SignedPower=off  SaturateOnIntegerOverflow=on
  Math Function1 : Math  Operator=rem  SignedPower=off  SaturateOnIntegerOverflow=on
  Switch1 : Switch  Criteria=u2 > Threshold
  Switch10 : Switch  Criteria=u2 ~= 0  Threshold=360
  Switch11 : Switch  Criteria=u2 ~= 0  Threshold=360
  Switch7 : Switch  Criteria=u2 > Threshold  Threshold=360
  Switch8 : Switch  Criteria=u2 ~= 0  Threshold=360
  Switch9 : Switch  Criteria=u2 > Threshold
  Unary Minus1 : UnaryMinus
  Out1 : Outport
  wires:
  Logical Operator1/1 -> Switch10/2
  Compare To Constant8/1 -> Logical Operator1/2
  Compare To Constant7/1 -> Logical Operator1/1
  Switch9/1 -> Out1/1
  Switch11/1 -> Switch9/3
  Constant11/1 -> Add12/1
  Add12/1 -> Switch11/3
  Unary Minus1/1 -> Switch11/1
  Constant5/1 -> Add11/2
  Add11/1 -> Unary Minus1/1
  Compare To Constant6/1 -> Switch11/2
  Constant4/1 -> Add10/1
  Add10/1 -> Switch10/3
  Constant2/1 -> Add9/1
  Add9/1 -> Switch10/1
  Switch10/1 -> Switch9/1
  Switch1/1 -> Switch9/2, Add10/2, Compare To Constant8/1, Compare To Constant7/1, Add9/2, Compare To Constant6/1, Add12/2, Add11/1
  Math Function1/1 -> Switch8/1
  Compare To Constant5/1 -> Switch8/2
  Switch8/1 -> Switch1/3
  Constant1/1 -> Math Function/2, Math Function1/2
  Math Function/1 -> Switch7/1
  Switch7/1 -> Switch1/1
  In1/1 -> Switch7/3, Switch7/2, Math Function/1, Math Function1/1, Compare To Constant5/1, Switch8/3, Switch1/2

== system MPC2018a/Lateral_Control_Simulation-2/Vehicle Model ==
  SteerCmd : Inport
  AccelCmd : Inport  Port=2
  DecelCmd : Inport  Port=3
  Direction : Inport  Port=4
  Acceleration to Velocity : Subsystem  TreatAsAtomicUnit=on
  Constant5 : Constant  Value=4  SampleTime=-1
  Degrees to Radians : simulink_extras/Transformations/Degrees to Radians
  Delayed Steering System : Subsystem
  Kinematic Steering : vehdynlibsteering/Kinematic Steering  StrgType=Ackerman  StrgRatioType=Constant  Loc=Front  NrmlFctr=1  TrckWdth=2.35  WhlBase=5.275  Db=0  StrgRng=1.25*pi  StrgAngBpts="[-6.2832   -5.0265   -3.7699   -2.5133   -1.2566         0    1.2566    2.5133    3.7699    5.0265    6.2832]"  StrgRatioTbl=|  StrgRatio=1  StrgArmLngth=0.1  RckCsLngth=0.5  TieRodLngth=0.248  D=0.2  PnnRadius=0.0057  PnnRadiusTbl="[0.0055    0.0055    0.0056    0.0057    0.0058    0.0057    0.0057    0.0057    0.0056    0.0055    0.0055]"  RodLngth=0.1  ParaArmLngth=0.9  aMode=2
      | [13.5000   13.3750   13.2500   13.1250   13.0000   13.0000   13.0000   13.1250   13.2500   13.3750   13.5000
      | ]
  Mux : Mux  Inputs=2
  Subsystem : Subsystem
  Terminator : Terminator
  Terminator1 : Terminator
  Terminator2 : Terminator
  Vehicle Body 3DOF Dual Track : autolibshared/Vehicle Body 3DOF Single Track  trackMode=Dual  inputMode=External longitudinal velocity  frontSteerMode=on  rearSteerMode=off  windMode=off  muMode=off  extFMode=off  extMMode=off  extXo=off  extpsio=off  extxdoto=off  extro=off  extYo=off  extTamb=off  extydoto=off  aMode=2  NF=2  NR=4  m=2400  a=1.45  b=1.45  h=0.8  X_o=startPose(1)+cosd(startPose(3))*1.6  xdot_o=0  CalphaMode=off  sigmaMode=off  d=0  w=[1.9,1.9]  Cy_f=155494.663  Cy_r=155494.663  sigma_f=.1  sigma_r=.1  alpha_f_brk=[-.1 .1]  Cy_f_data=[-9e3 9e3]  alpha_r_brk=[-.1 .1]  Cy_r_data=[-9e3 9e3]  Y_o=startPose(2) +sind(startPose(3))*1.6  ydot_o=0  Izz=5046  psi_o=deg2rad(startPose(3))  r_o=0  Af=6  Cd=.3  Cl=0  Cpm=.1  beta_w=[0:0.01:0.3]  Cs=[0:0.03:0.9]  Cym=[0:0.01:0.3]  Pabs=101325  Tair=273  g=9.81  mu=1  xdot_tol=.01  Fznom=5000  Fxtire_sat=7e4  Fytire_sat=7e4  longOff=0  latOff=0  vertOff=0  wrapAng=off
      settings: SourceProductBaseCode=PW,MT,VE,VP
  VehicleInfo : Outport  VectorParamsAs1DForOutWhenUnconnected=off
  Out1 : Outport  Port=2
  wires:
  Direction/1 -> Acceleration to Velocity/3(Direction), Subsystem/7(<Direction>)
  SteerCmd/1 -> Delayed Steering System/1(SteerCmd)  "CurrSteer"
  DecelCmd/1 -> Acceleration to Velocity/2(DecelCmd)
  AccelCmd/1 -> Acceleration to Velocity/1(AccelCmd)
  Subsystem/1(VehicleInfo) -> VehicleInfo/1
  Vehicle Body 3DOF Dual Track/1 -> Subsystem/2(Info)
  Vehicle Body 3DOF Dual Track/2 -> Subsystem/3(In3)
  Vehicle Body 3DOF Dual Track/3 -> Subsystem/4(In4)
  Vehicle Body 3DOF Dual Track/4 -> Subsystem/5(In5)
  Vehicle Body 3DOF Dual Track/5 -> Subsystem/6(In6)
  Vehicle Body 3DOF Dual Track/6 -> Terminator/1
  Vehicle Body 3DOF Dual Track/7 -> Terminator1/1
  Kinematic Steering/1 -> Terminator2/1
  Kinematic Steering/2 -> Mux/1
  Kinematic Steering/3 -> Mux/2
  Degrees to Radians/1 -> Kinematic Steering/1
  Delayed Steering System/1(CurrSteer) -> Out1/1, Subsystem/1(CurrSteer), Degrees to Radians/1  "CurrSteer"
  Mux/1 -> Vehicle Body 3DOF Dual Track/1
  Constant5/1 -> Vehicle Body 3DOF Dual Track/2

== system MPC2018a/Lateral_Control_Simulation-2/simulation_stop ==
  In1 : Inport
  In2 : Inport  Port=2
  Compare To Constant : simulink/Logic and Bit Operations/Compare To Constant  relop=<=  const=-320  OutDataTypeStr=boolean
  Compare To Constant1 : simulink/Logic and Bit Operations/Compare To Constant  relop=>=  const=-340  OutDataTypeStr=boolean
  Compare To Constant2 : simulink/Logic and Bit Operations/Compare To Constant  relop=<=  const=240  OutDataTypeStr=boolean
  Compare To Constant3 : simulink/Logic and Bit Operations/Compare To Constant  relop=>=  const=220  OutDataTypeStr=boolean
  Logical Operator : Logic  AllPortsSameDT=off  OutDataTypeStr=boolean
  Logical Operator1 : Logic  AllPortsSameDT=off  OutDataTypeStr=boolean
  Logical Operator2 : Logic  AllPortsSameDT=off  OutDataTypeStr=boolean
  Stop Simulation : Stop
  wires:
  Logical Operator1/1 -> Stop Simulation/1
  Compare To Constant/1 -> Logical Operator/1
  In1/1 -> Compare To Constant/1, Compare To Constant1/1
  Compare To Constant1/1 -> Logical Operator/2
  Logical Operator/1 -> Logical Operator1/1
  Logical Operator2/1 -> Logical Operator1/2
  Compare To Constant2/1 -> Logical Operator2/1
  Compare To Constant3/1 -> Logical Operator2/2
  In2/1 -> Compare To Constant2/1, Compare To Constant3/1

== system MPC2018a/Lateral_Control_Simulation-1/Vehicle Model/Acceleration to Velocity ==
  AccelCmd : Inport  PortDimensions=[1 1]
  DecelCmd : Inport  Port=2  PortDimensions=[1 1]
  Direction : Inport  Port=3
  AND : Logic  IconShape=distinctive  AllPortsSameDT=off  OutDataTypeStr=boolean
  Abs : Abs
  Add : Sum  Inputs=+-
  Compare To Zero : simulink/Logic and Bit Operations/Compare To Zero  relop=<=  OutDataTypeStr=boolean
  Compare To Zero1 : simulink/Logic and Bit Operations/Compare To Zero  relop=>  OutDataTypeStr=boolean
  Constant : Constant  Value=0.05
  Constant1 : Constant  Value=0
  Minus : Sum  Inputs=+-
  Product1 : Product
  Saturated integrator : Integrator  ExternalReset=either  LimitOutput=on  LowerSaturationLimit=0  AbsoluteTolerance=1e-3  ZeroCross=off
  Switch : Switch  Criteria=u2 > Threshold
  Unit Delay : UnitDelay  SampleTime=-1  HasFrameUpgradeWarning=on
  Velocity : Outport  VectorParamsAs1DForOutWhenUnconnected=off
  wires:
  Direction/1 -> Product1/2, Saturated integrator/2
  AccelCmd/1 -> Add/1
  Add/1 -> Saturated integrator/1
  DecelCmd/1 -> Compare To Zero1/1, Add/2
  Unit Delay/1 -> Abs/1
  Abs/1 -> Minus/1
  Constant/1 -> Minus/2
  Minus/1 -> Compare To Zero/1
  Compare To Zero/1 -> AND/2
  Compare To Zero1/1 -> AND/1
  AND/1 -> Switch/2  "Reset velocity to zero"
  Switch/1 -> Unit Delay/1, Velocity/1
  Constant1/1 -> Switch/1
  Saturated integrator/1 -> Product1/1
  Product1/1 -> Switch/3

== system MPC2018a/Lateral_Control_Simulation-1/Vehicle Model/Delayed Steering System ==
  SteerCmd : Inport
  Add : Sum  Inputs=+-
  Constant : Constant  Value=0
  Delay : TransferFcn  Denominator=[0.1 0]
  Sum : Sum  Inputs=|++
  CurrSteer : Outport  VectorParamsAs1DForOutWhenUnconnected=off
  wires:
  Add/1 -> Delay/1
  SteerCmd/1 -> Sum/1
  Delay/1 -> Add/2
  Sum/1 -> CurrSteer/1
  Constant/1 -> Sum/2

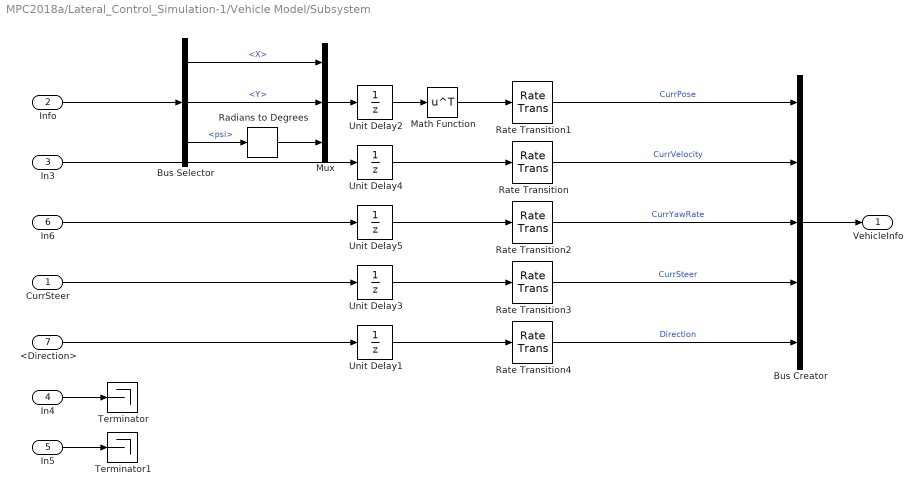
== system MPC2018a/Lateral_Control_Simulation-1/Vehicle Model/Subsystem ==
  CurrSteer : Inport
  Info : Inport  Port=2
  In3 : Inport  Port=3
  In4 : Inport  Port=4
  In5 : Inport  Port=5
  In6 : Inport  Port=6
  <Direction> : Inport  Port=7
  Bus Creator : BusCreator  Inputs=5
  Bus Selector : BusSelector  OutputSignals=InertFrm.Geom.Disp.X,InertFrm.Geom.Disp.Y,InertFrm.Cg.Ang.psi
  Math Function : Math  Operator=transpose  SaturateOnIntegerOverflow=on
  Mux : Mux  Inputs=3
  Radians to Degrees : simulink_extras/Transformations/Radians to Degrees
  Rate Transition : RateTransition  OutPortSampleTime=0.05
  Rate Transition1 : RateTransition  InitialCondition=startPose  OutPortSampleTime=0.05
  Rate Transition2 : RateTransition  OutPortSampleTime=0.05
  Rate Transition3 : RateTransition  OutPortSampleTime=0.05
  Rate Transition4 : RateTransition  InitialCondition=1  OutPortSampleTime=0.05
  Terminator : Terminator
  Terminator1 : Terminator
  Unit Delay1 : UnitDelay  InitialCondition=1  SampleTime=-1  HasFrameUpgradeWarning=on
  Unit Delay2 : UnitDelay  InitialCondition=startPose  SampleTime=-1  HasFrameUpgradeWarning=on
  Unit Delay3 : UnitDelay  SampleTime=-1  HasFrameUpgradeWarning=on
  Unit Delay4 : UnitDelay  SampleTime=-1  HasFrameUpgradeWarning=on
  Unit Delay5 : UnitDelay  SampleTime=-1  HasFrameUpgradeWarning=on
  VehicleInfo : Outport  VectorParamsAs1DForOutWhenUnconnected=off
  wires:
  Unit Delay1/1 -> Rate Transition4/1
  CurrSteer/1 -> Unit Delay3/1
  Unit Delay5/1 -> Rate Transition2/1
  <Direction>/1 -> Unit Delay1/1
  Unit Delay4/1 -> Rate Transition/1
  Math Function/1 -> Rate Transition1/1
  Rate Transition/1 -> Bus Creator/2  "CurrVelocity"
  Unit Delay3/1 -> Rate Transition3/1
  Rate Transition3/1 -> Bus Creator/4  "CurrSteer"
  Rate Transition1/1 -> Bus Creator/1  "CurrPose"
  Rate Transition2/1 -> Bus Creator/3  "CurrYawRate"
  Rate Transition4/1 -> Bus Creator/5  "Direction"
  In5/1 -> Terminator1/1
  Unit Delay2/1 -> Math Function/1
  Info/1 -> Bus Selector/1
  Radians to Degrees/1 -> Mux/3
  Bus Selector/2 -> Mux/2  "<Y>"
  Bus Selector/1 -> Mux/1  "<X>"
  Mux/1 -> Unit Delay2/1
  In3/1 -> Unit Delay4/1
  In4/1 -> Terminator/1
  In6/1 -> Unit Delay5/1
  Bus Selector/3 -> Radians to Degrees/1  "<psi>"
  Bus Creator/1 -> VehicleInfo/1

== system MPC2018a/Lateral_Control_Simulation-1/preview_dis_caculation/far_pre_dis caculaiton ==
  vehiclespeed : Inport
  pre_time : Inport  Port=2
  pre_base : Inport  Port=3
  param : Inport  Port=4
  Add : Sum
  Add1 : Sum
  MinMax : MinMax  Function=max  Inputs=2
  Product : Product
  farprepointdis : Outport
  wires:
  MinMax/1 -> farprepointdis/1
  Add1/1 -> MinMax/2
  Add/1 -> MinMax/1
  param/1 -> Add1/2
  pre_base/1 -> Add/2, Add1/1
  Product/1 -> Add/1
  pre_time/1 -> Product/2
  vehiclespeed/1 -> Product/1

== system MPC2018a/Lateral_Control_Simulation-1/preview_dis_caculation/near_pre_dis caculaiton ==
  vehiclespeed : Inport
  Add : Sum
  Add1 : Sum
  Constant3 : Constant  Value=1.5  OutDataTypeStr=single
  MinMax : MinMax  Function=max  Inputs=2
  Product : Product
  pre_base : Constant  Value=2  OutDataTypeStr=single
  pre_time : Constant  Value=2  OutDataTypeStr=single
  nearprepointdis : Outport
  wires:
  vehiclespeed/1 -> Product/1
  pre_time/1 -> Product/2
  Product/1 -> Add/1
  pre_base/1 -> Add1/1, Add/2
  Constant3/1 -> Add1/2
  Add/1 -> MinMax/1
  Add1/1 -> MinMax/2
  MinMax/1 -> nearprepointdis/1

== system MPC2018a/Lateral_Control_Simulation-2/Vehicle Model/Acceleration to Velocity ==
  AccelCmd : Inport  PortDimensions=[1 1]
  DecelCmd : Inport  Port=2  PortDimensions=[1 1]
  Direction : Inport  Port=3
  AND : Logic  IconShape=distinctive  AllPortsSameDT=off  OutDataTypeStr=boolean
  Abs : Abs
  Add : Sum  Inputs=+-
  Compare To Zero : simulink/Logic and Bit Operations/Compare To Zero  relop=<=  OutDataTypeStr=boolean
  Compare To Zero1 : simulink/Logic and Bit Operations/Compare To Zero  relop=>  OutDataTypeStr=boolean
  Constant : Constant  Value=0.05
  Constant1 : Constant  Value=0
  Minus : Sum  Inputs=+-
  Product1 : Product
  Saturated integrator : Integrator  ExternalReset=either  LimitOutput=on  LowerSaturationLimit=0  AbsoluteTolerance=1e-3  ZeroCross=off
  Switch : Switch  Criteria=u2 > Threshold
  Unit Delay : UnitDelay  SampleTime=-1  HasFrameUpgradeWarning=on
  Velocity : Outport  VectorParamsAs1DForOutWhenUnconnected=off
  wires:
  Direction/1 -> Product1/2, Saturated integrator/2
  AccelCmd/1 -> Add/1
  Add/1 -> Saturated integrator/1
  DecelCmd/1 -> Compare To Zero1/1, Add/2
  Unit Delay/1 -> Abs/1
  Abs/1 -> Minus/1
  Constant/1 -> Minus/2
  Minus/1 -> Compare To Zero/1
  Compare To Zero/1 -> AND/2
  Compare To Zero1/1 -> AND/1
  AND/1 -> Switch/2  "Reset velocity to zero"
  Switch/1 -> Unit Delay/1, Velocity/1
  Constant1/1 -> Switch/1
  Saturated integrator/1 -> Product1/1
  Product1/1 -> Switch/3

== system MPC2018a/Lateral_Control_Simulation-2/Vehicle Model/Delayed Steering System ==
  SteerCmd : Inport
  Add : Sum  Inputs=+-
  Constant : Constant  Value=0
  Delay : TransferFcn  Denominator=[0.1 0]
  Sum : Sum  Inputs=|++
  CurrSteer : Outport  VectorParamsAs1DForOutWhenUnconnected=off
  wires:
  Add/1 -> Delay/1
  Delay/1 -> Add/2
  Constant/1 -> Sum/2
  SteerCmd/1 -> Sum/1
  Sum/1 -> CurrSteer/1

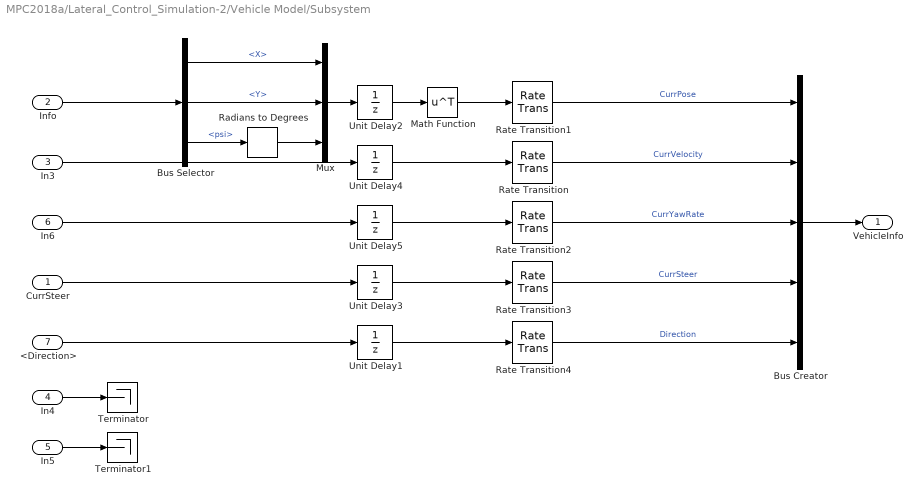
== system MPC2018a/Lateral_Control_Simulation-2/Vehicle Model/Subsystem ==
  CurrSteer : Inport
  Info : Inport  Port=2
  In3 : Inport  Port=3
  In4 : Inport  Port=4
  In5 : Inport  Port=5
  In6 : Inport  Port=6
  <Direction> : Inport  Port=7
  Bus Creator : BusCreator  Inputs=5
  Bus Selector : BusSelector  OutputSignals=InertFrm.Geom.Disp.X,InertFrm.Geom.Disp.Y,InertFrm.Cg.Ang.psi
  Math Function : Math  Operator=transpose  SaturateOnIntegerOverflow=on
  Mux : Mux  Inputs=3
  Radians to Degrees : simulink_extras/Transformations/Radians to Degrees
  Rate Transition : RateTransition  OutPortSampleTime=0.05
  Rate Transition1 : RateTransition  InitialCondition=startPose  OutPortSampleTime=0.05
  Rate Transition2 : RateTransition  OutPortSampleTime=0.05
  Rate Transition3 : RateTransition  OutPortSampleTime=0.05
  Rate Transition4 : RateTransition  InitialCondition=1  OutPortSampleTime=0.05
  Terminator : Terminator
  Terminator1 : Terminator
  Unit Delay1 : UnitDelay  InitialCondition=1  SampleTime=-1  HasFrameUpgradeWarning=on
  Unit Delay2 : UnitDelay  InitialCondition=startPose  SampleTime=-1  HasFrameUpgradeWarning=on
  Unit Delay3 : UnitDelay  SampleTime=-1  HasFrameUpgradeWarning=on
  Unit Delay4 : UnitDelay  SampleTime=-1  HasFrameUpgradeWarning=on
  Unit Delay5 : UnitDelay  SampleTime=-1  HasFrameUpgradeWarning=on
  VehicleInfo : Outport  VectorParamsAs1DForOutWhenUnconnected=off
  wires:
  Unit Delay1/1 -> Rate Transition4/1
  CurrSteer/1 -> Unit Delay3/1
  Unit Delay5/1 -> Rate Transition2/1
  <Direction>/1 -> Unit Delay1/1
  Unit Delay4/1 -> Rate Transition/1
  Math Function/1 -> Rate Transition1/1
  Rate Transition/1 -> Bus Creator/2  "CurrVelocity"
  Unit Delay3/1 -> Rate Transition3/1
  Rate Transition3/1 -> Bus Creator/4  "CurrSteer"
  Rate Transition1/1 -> Bus Creator/1  "CurrPose"
  Rate Transition2/1 -> Bus Creator/3  "CurrYawRate"
  Rate Transition4/1 -> Bus Creator/5  "Direction"
  In5/1 -> Terminator1/1
  Unit Delay2/1 -> Math Function/1
  Info/1 -> Bus Selector/1
  Radians to Degrees/1 -> Mux/3
  Bus Selector/2 -> Mux/2  "<Y>"
  Bus Selector/1 -> Mux/1  "<X>"
  Mux/1 -> Unit Delay2/1
  In3/1 -> Unit Delay4/1
  In4/1 -> Terminator/1
  In6/1 -> Unit Delay5/1
  Bus Selector/3 -> Radians to Degrees/1  "<psi>"
  Bus Creator/1 -> VehicleInfo/1

== matlab function MPC2018a/Lateral_Control_Simulation-1/path_process ==
  data: curpoint input; d output; key_x output; key_y output; key_theta output; R output; dis_last output; pre_dis_far input; prepointcount_far output; m_angle_head output; m_angle_point output; pre_x output; pre_y output; key_angle_error output; pre_dis_near input; curvehhead input; two_preview_on input; v_tra output
function [d,key_x,key_y,key_theta,R,dis_last,prepointcount_far,m_angle_head,m_angle_point,pre_x,pre_y,key_angle_error,v_tra]  = fcn(curpoint,pre_dis_far,pre_dis_near,curvehhead,two_preview_on)
Q = load('NewBaiYunPathDown6_13.mat');
dis_last = 100000;
abc=1;
abc_last = 1;
n=1;
x0=0;
y0=0;
lng0 = Q.BaiYunEmpty(2,1);
lat0 = Q.BaiYunEmpty(1,1);
temp_n = length(Q.BaiYunEmpty(1,:));
while (n<temp_n)    
lng2 = Q.BaiYunEmpty(2,n);
lat2 = Q.BaiYunEmpty(1,n);
temp_x=(lng2-lng0)*111700*cos(lat2/180*pi);
temp_y=(lat2-lat0)*111700;    
x1 = x0 + temp_x;
y1 = y0 + temp_y;
x2=curpoint(1);
y2=curpoint(2);
    dis=sqrt((x1-x2)^2+(y1-y2)^2);
    if(dis<dis_last)
        abc=n;
        dis_last = dis;
    else
        abc=abc_last;
    end
abc_last = abc;
n = n+1;
end
keypointlist = abc;
key_x=(Q.BaiYunEmpty(2,keypointlist)-lng0)*111700*cos(Q.BaiYunEmpty(1,keypointlist)/180*pi);
key_y=(Q.BaiYunEmpty(1,keypointlist)-lat0)*111700; 
key_theta=Q.BaiYunEmpty(3,keypointlist);
key_x1=(Q.BaiYunEmpty(2,keypointlist+1)-lng0)*111700*cos(Q.BaiYunEmpty(1,keypointlist+1)/180*pi);
key_y1=(Q.BaiYunEmpty(1,keypointlist+1)-lat0)*111700; 
key_delta_x = key_x - curpoint(1);
key_delta_y = key_y - curpoint(2);
key_delta_x1 = key_x1 - curpoint(1);
key_delta_y1 = key_y1 - curpoint(2);
dis1 = sqrt((key_delta_x1)^2+(key_delta_y1)^2);
dis2 = sqrt((key_x1-key_x)^2+(key_y1-key_y)^2);
area = 1/4*sqrt((dis_last+dis1+dis2)*(dis_last+dis1-dis2)*(dis_last+dis2-dis1)*(dis1+dis2-dis_last));
if(dis2>=0.01)
    d=2.0*area/dis2;
else
    d=dis_last;
end       
if(key_delta_x>-0.0001&&key_delta_x<0.0001)
    if(key_delta_y>0)
        key_point_direction=0;
    else
        key_point_direction=180;
    end    
else    
   key_point_direction = atan(key_delta_y / key_delta_x) / pi*180;
    if (key_delta_x > 0) 
        key_point_direction = 90 - key_point_direction;
    else
        key_point_direction = 270 - key_point_direction;
    end
end
%%%%%%%%%%%%%%%%%%%%%%%%%%%%%%%%%%%%%%%%%%%%%%%%%%%%%%%%%%%%%%%%%%%%%%%%%%%%%%%%%%%%%%%%%%%%%%%%%%%%%
subdis_far=0;
prepointcount_far = 0;
prepointcount_near = 0;
while(subdis_far<pre_dis_far&&keypointlist+prepointcount_far<temp_n)    
    lng3 = Q.BaiYunEmpty(2,keypointlist+prepointcount_far);
    lng4 = Q.BaiYunEmpty(2,keypointlist+prepointcount_far+1);
    lat3 = Q.BaiYunEmpty(1,keypointlist+prepointcount_far);
    lat4 = Q.BaiYunEmpty(1,keypointlist+prepointcount_far+1);    
    d_x=(lng4-lng3)*111700*cos(lat4/180*pi);
    d_y=(lat4-lat3)*111700;    
    iDistance = sqrt(d_x^2+d_y^2);
    subdis_far = subdis_far+iDistance;
    if(two_preview_on)
        if(subdis_far>=pre_dis_near)
            prepointcount_near = prepointcount_far;
        else
            prepointcount_near = 0;
        end
    end
    prepointcount_far = prepointcount_far+1;
end
theta_veh = curvehhead;
k=min(keypointlist+prepointcount_far,temp_n);
temp1=Q.BaiYunEmpty(3,k);
temp2=Q.BaiYunEmpty(3,keypointlist+10);
m_angle_head = -(temp1-theta_veh);
key_angle_error = -(temp2-theta_veh);
if (m_angle_head > 180) 
   m_angle_head = m_angle_head - 360;       
elseif(m_angle_head < -180) 
   m_angle_head = m_angle_head + 360;
end
if (key_angle_error > 180) 
   key_angle_error = key_angle_error - 360;       
elseif(key_angle_error < -180) 
   key_angle_error = key_angle_error + 360;
end
%%%%%%%%%%%%%%%%%%%%%%%%%%%%%%%%%%%%%%%%%%%%%%%%%%%%%%%%%%%%%%%%%%%%%%%%%%%%%%%%%%%%%%%%%%%%
temp3=Q.BaiYunEmpty(3,keypointlist+50);
temp4=Q.BaiYunEmpty(3,keypointlist+51);
temp_angle_error = -(temp4 - temp3);
if (temp_angle_error > 180) 
   temp_angle_error = temp_angle_error - 360;       
elseif(temp_angle_error < -180) 
   temp_angle_error = temp_angle_error + 360;
end
temp_angle_error=temp_angle_error/2;
lng6 = Q.BaiYunEmpty(2,keypointlist+50);
lng7 = Q.BaiYunEmpty(2,keypointlist+51);
lat6 = Q.BaiYunEmpty(1,keypointlist+52);
lat7 = Q.BaiYunEmpty(1,keypointlist+51);    
dx2=(lng7-lng6)*111700*cos(lat7/180*pi);
dy2=(lat7-lat6)*111700;    
ds = sqrt(dx2^2+dy2^2);
ds=ds/2;
R=ds/sin(abs(temp_angle_error));
% rou = 1/R;
% theta_tra = atan(5.275/R);
% if(temp_angle_error<0)
%     theta_tra = -theta_tra;
% end
% theta_tra=0;
%%%%%%%%%%%%%%%%%%%%%%%%%%%%%%%%%%%%%%%%%%%%%%%%%%%%%%%%%%%%%%%%%%%%%%%%%%%%%%%%%%%%%%%%
if(two_preview_on)
    prepointcount = prepointcount_near;
else
    prepointcount = prepointcount_far;
end

lng5 = Q.BaiYunEmpty(2,keypointlist+prepointcount);
lat5 = Q.BaiYunEmpty(1,keypointlist+prepointcount);

d_x_1=(lng5-lng0)*111700*cos(lat0/180*pi);
d_y_1=(lat5-lat0)*111700;    

dx_far=d_x_1-curpoint(1);
dy_far=d_y_1-curpoint(2);

dx = dx_far;
dy = dy_far;
temp3 = curvehhead;

if(dx>-0.0001&&dx<0.0001)
    if(dy>0)
        pre_point_direction=0;
    else
        pre_point_direction=180;
    end
else
   pre_point_direction = atan(dy / dx) / pi*180;
    if (dx > 0) 
        pre_point_direction = 90 - pre_point_direction;
    else
        pre_point_direction = 270 - pre_point_direction;
    end
end        
m_angle_point = -(pre_point_direction - curvehhead);
    if (m_angle_point > 180)
        m_angle_point = m_angle_point - 360;
    else
        if (m_angle_point < -180)
         m_angle_point = m_angle_point + 360;
        end
    end

near_angle=pre_point_direction-key_point_direction;

if (near_angle > 180)
    near_angle = near_angle - 360;
end
if (near_angle < -180)
    near_angle = near_angle + 360;
end
if(near_angle>0)
    d=-d;
end

pre_x=d_x_1;
pre_y=d_y_1;

% v_tra = Q.BaiYunEmpty(4,keypointlist+prepointcount)*3.6;
v_tra = 3;
end
